simulink model "test"  (R2016a)
settings: Solver=VariableStepAuto  StartTime=0.0  StopTime=10.0  RelTol=1e-3
settings Model: Creator=mrlisdim  LastModifiedBy=mrlisdim

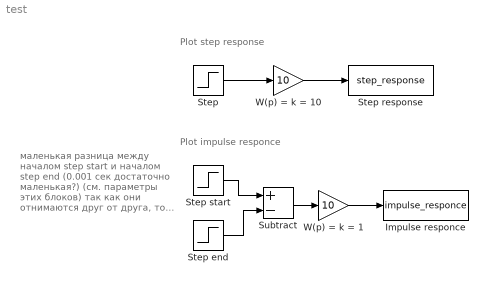
== system test ==
  note: маленькая разница
      | между началом step start
      | и началом step end
      | (0.001 сек достаточно
      | маленькая?)
      | (см. параметры этих блоков)
      |
      | так как они отнимаются друг
      | от друга, то получаем типа
      | импульс
  note: Plot impulse responce
  note: Plot step response
  Impulse responce : ToWorkspace  VariableName=impulse_responce  SaveFormat=Timeseries  SampleTime=-1
  Step : Step  Time=0  SampleTime=0
  Step end : Step  Time=1.001  After=100  SampleTime=0
  Step response : ToWorkspace  VariableName=step_response  SaveFormat=Timeseries  SampleTime=-1
  Step start : Step  After=100  SampleTime=0
  Subtract : Sum  Inputs=+-
  W(p) = k = 1 : Gain  Gain=10
  W(p) = k = 10 : Gain  Gain=10
  wires:
  Step/1 -> W(p) = k = 10/1
  W(p) = k = 10/1 -> Step response/1
  Step start/1 -> Subtract/1
  Step end/1 -> Subtract/2
  Subtract/1 -> W(p) = k = 1/1
  W(p) = k = 1/1 -> Impulse responce/1
